simulink model "Senorless"  (R2023a)
settings: Solver=FixedStepDiscrete  StartTime=0.0  StopTime=5  FixedStep=1/FOC_FRQ  RelTol=1e-3
values from neighbouring files (symbols this model uses):
  ADC_REF = 3.6    [Senorless.sldd]
  ADC_SAMPLE_MAX = 32767.0    [Senorless.sldd]
  AMP_GAIN = 16.0    [Senorless.sldd]
  CURR_INPUT = 3276.0    [Senorless.sldd]
  CURR_KI = 380.0    [Senorless.sldd]
  CURR_KP = 0.04    [Senorless.sldd]
  CURR_LIMIT = 0.95    [Senorless.sldd]
  CURR_OVER = 6.0    [Senorless.sldd]
  CURR_POINT_GAIN = 7.0    [Senorless.sldd]
  CURR_STEP = 32760.0    [Senorless.sldd]
  CURR_UNDER = 0.03    [Senorless.sldd]
  CURR_WIDTH = 6552.0    [Senorless.sldd]
  FOC_FRQ = 25000.0    [Senorless.sldd]
  GAMMA = 32767.0    [Senorless.sldd]
  IMAX = 10.0    [Senorless.sldd]
  LPF_FRQ = 2000.0    [Senorless.sldd]
  MOTOR_DAMPER = 2.06E-7    [Senorless.sldd]
  MOTOR_FLUX = 0.00212352    [Senorless.sldd]
  MOTOR_INERTIA = 4.0E-7    [Senorless.sldd]
  MOTOR_LS = 0.000536    [Senorless.sldd]
  MOTOR_PN = 7.0    [Senorless.sldd]
  MOTOR_RS = 4.0    [Senorless.sldd]
  OPEN_IQ = 0.28    [Senorless.sldd]
  OPEN_IQ_MIN = 0.05    [Senorless.sldd]
  OPEN_IQ_SLOW = 0.1    [Senorless.sldd]
  OPEN_SPD = 1000.0    [Senorless.sldd]
  OPEN_SPD_SLOW = 180.0    [Senorless.sldd]
  OPEN_TIME = 0.5    [Senorless.sldd]
  OPEN_TIME_NFO = 0.5    [Senorless.sldd]
  PLL_LIMIT = 0.9    [Senorless.sldd]
  PLL_WIDTH = 800.0    [Senorless.sldd]
  PWM_FRQ = 96000000.0    [Senorless.sldd]
  RS_HUNT = 0.02    [Senorless.sldd]
  SMOK_FRQ = 600.0    [Senorless.sldd]
  SPD_LIMIT = 0.9    [Senorless.sldd]
  SPD_LPF_LEVEL = 0.0    [Senorless.sldd]
  SPD_MAX = 12000.0    [Senorless.sldd]
  SPD_MIN = 4000.0    [Senorless.sldd]
  SPD_REDUCE = 380.0    [Senorless.sldd]
  SPD_STEP = 6.0    [Senorless.sldd]
  SPD_WIDTH = 20.0    [Senorless.sldd]
  THETA_ERR_LIMIT = 8192.0    [Senorless.sldd]
  TS_POINT_GAIN = 10.0    [Senorless.sldd]
  UDC = 48.0    [Senorless.sldd]
  UDC_GAIN = 21.0    [Senorless.sldd]
  UDC_POINT_GAIN = 10.0    [Senorless.sldd]
undefined symbols (not defined in the file or in its folder): curr_q_ki, curr_q_kp, DiscIntNeverNeededParam, magnitude, PLL_LPF_LEVEL, Udc
libraries: simulink x20, slpidlib x5, mcbcontrolslib x2, mcbplantlib x1, autolibpmsmexterior x1, spspowerguiLib x1
(part 3 of 8)

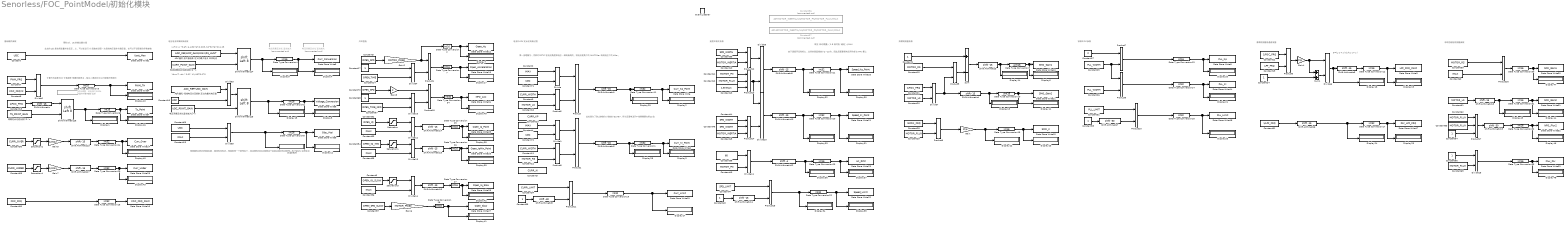
== system Senorless/FOC_PointModel/初始化模块 ==
  note: 非线性磁链观测器参数
  note: 由于速度环没有标幺，出来的是直接放大2^15的，因此后面要把电流环的标幺IMAX算上
  note: 带宽*转动惯量/（1.5*极对数*磁链）/IMAX
  note: 速度环相关系数
  note: 滑模观测器低通滤波器
  note: 锁相环PID参数
  note: 观测器电流电压转换系数，指将电压电流转换到同一个参考系下，如这里电压定点值乘这个后就会换去电流参考：32768/10这种定点
  note: 滑模观测器系数
  note: 开环强拖
  note: 电流环KPKI定点化转换过程
  note: 基础硬件参数
  note: 电压电流采集转换系数
  note: 此处的Udc是全局变量并非宏定义，可以在运行init函数前读取一次母线电压值作为确定值，也可以不读取修改字典参数
  note: 此处是为了防止参数为小数放大32767，所以后面电流环PI结果需要左移15位
  note: 第一部理解为，同样的32767在电流角度和电压角度是不一样的概念，这里是做转换用的，将电流视角下的MAX=IMax转到电压下的UMax。
  note: 限制Ud、Uq的输出最大值
  note: iwf = iw *3.6f / 6.4/32767/0.005 /10*32767=11.25
  note: Vbus = vdc * 3.6f * 41/48=3.075
  note: 计算方式就是PWM计数频率/想要的频率/2，除以二是因为中心计数模式导致的
  note: a=(ω c​ T s​ )/(1+ω c​ T s​ )
  ADC量程*母线电压分压倍数/定义的最大电压值 : Constant  Value=ADC_REF*UDC_GAIN
  ADC量程/放大器倍数/定义的最大电流/采样电流 : Constant  Value=ADC_REF/AMP_GAIN/IMAX/RS_HUNT
  Constant{,69,71..72} (4 alike) : Constant  Value=UDC  OutDataTypeStr=int16
  Constant{1,17,24,33,35,48,68} (7 alike) : Constant  OutDataTypeStr=single
  Constant10 : Constant  Value=MOTOR_LS  OutDataTypeStr=single
  Constant11 : Constant  Value=CURR_WIDTH  OutDataTypeStr=single
  Constant12 : Constant  Value=MOTOR_RS  OutDataTypeStr=single
  Constant13 : Constant  Value=IMAX  OutDataTypeStr=single
  Constant14 : Constant  Value=OPEN_TIME
  Constant15 : Constant  Value=MOTOR_RS  OutDataTypeStr=single
  Constant16 : Constant  Value=UDC
  Constant18 : Constant  Value=1/FOC_FRQ  VectorParams1D=off  OutDataTypeStr=double
  Constant19 : Constant  Value=LPF_FRQ
  Constant2 : Constant  Value=IMAX  OutDataTypeStr=single
  Constant20 : Constant  Value=MOTOR_LS  OutDataTypeStr=single
  Constant21 : Constant  Value=1/FOC_FRQ  VectorParams1D=off  OutDataTypeStr=double
  Constant22 : Constant  Value=1/FOC_FRQ  VectorParams1D=off  OutDataTypeStr=double
  Constant23 : Constant  Value=CURR_KP  OutDataTypeStr=single
  Constant25 : Constant  Value=PLL_WIDTH
  Constant26 : Constant  Value=PLL_WIDTH
  Constant27 : Constant  Value=2  OutDataTypeStr=single
  Constant28 : Constant  Value=SMOK_FRQ
  Constant{29,42,62..63,65} (5 alike) : Constant  Value=MOTOR_FLUX
  Constant3 : Constant  Value=CURR_KI  OutDataTypeStr=single
  Constant30 : Constant  Value=FOC_FRQ  VectorParams1D=off
  Constant31 : Constant  Value=1/LPF_FRQ  VectorParams1D=off  OutDataTypeStr=single
  Constant32 : Constant  Value=PLL_LIMIT
  Constant34 : Constant  Value=CURR_LIMIT  OutDataTypeStr=single
  Constant36 : Constant  Commented=on  Value=40*MOTOR_INERTIA/1.5/MOTOR_PN/MOTOR_FLUX/IMAX  OutDataTypeStr=single
  Constant37 : Constant  Commented=on  Value=40*40*MOTOR_INERTIA/1.5/MOTOR_PN/MOTOR_FLUX/IMAX  OutDataTypeStr=single
  Constant38 : Constant  Value=60  OutDataTypeStr=single
  Constant39 : Constant  Value=SPD_WIDTH
  Constant4 : Constant  Value=IMAX  OutDataTypeStr=single
  Constant40 : Constant  Value=MOTOR_INERTIA
  Constant41 : Constant  Value=MOTOR_PN
  Constant43 : Constant  Value=1.5*IMAX
  Constant44 : Constant  Value=SPD_WIDTH
  Constant45 : Constant  Value=MOTOR_INERTIA
  Constant46 : Constant  Value=SPD_WIDTH
  Constant47 : Constant  Value=SPD_LIMIT
  Constant49 : Constant  Value=MOTOR_PN
  Constant5 : Constant  Value=OPEN_SPD  OutDataTypeStr=single
  Constant50 : Constant  Value=CURR_OVER  VectorParams1D=off
  Constant52 : Constant  Value=OPEN_IQ
  Constant{53,55..56,60} (4 alike) : Constant  Value=IMAX
  Constant54 : Constant  Value=OPEN_IQ_MIN
  Constant57 : Constant  Value=OPEN_SPD_SLOW  OutDataTypeStr=single
  Constant58 : Constant  Value=CURR_UNDER  VectorParams1D=off
  Constant59 : Constant  Value=MOTOR_RS  OutDataTypeStr=single
  Constant6 : Constant  Value=OPEN_IQ_SLOW
  Constant61 : Constant  Value=MOTOR_LS  OutDataTypeStr=single
  Constant64 : Constant
  Constant66 : Constant
  Constant67 : Constant  Value=OPEN_TIME_NFO
  Constant7 : Constant  Value=PWM_FRQ
  Constant70 : Constant  Value=OPEN_SPD  OutDataTypeStr=single
  Constant8 : Constant  Value=FOC_FRQ*2  OutDataTypeStr=double
  Constant9 : Constant  Value=CURR_WIDTH  OutDataTypeStr=single
  Data Store Write : DataStoreWrite  DataStoreName=Curr_Kp_Point  IndexOptions=Index vector (dialog)  Indices=1  OutputSizes=1
  Data Store Write1 : DataStoreWrite  DataStoreName=Uout_Max  IndexOptions=Index vector (dialog)  Indices=1  OutputSizes=1
  Data Store Write10 : DataStoreWrite  DataStoreName=SMO_Gain1  IndexOptions=Index vector (dialog)  Indices=1  OutputSizes=1
  Data Store Write11 : DataStoreWrite  DataStoreName=SMO_Gain2  IndexOptions=Index vector (dialog)  Indices=1  OutputSizes=1
  Data Store Write12 : DataStoreWrite  DataStoreName=Open_Hz  IndexOptions=Index vector (dialog)  Indices=1  OutputSizes=1
  Data Store Write13 : DataStoreWrite  DataStoreName=Open_Acceleration  IndexOptions=Index vector (dialog)  Indices=1  OutputSizes=1
  Data Store Write14 : DataStoreWrite  DataStoreName=PLL_Ki  IndexOptions=Index vector (dialog)  Indices=1  OutputSizes=1
  Data Store Write15 : DataStoreWrite  DataStoreName=SMO_K  IndexOptions=Index vector (dialog)  Indices=1  OutputSizes=1
  Data Store Write16 : DataStoreWrite  DataStoreName=FOC_FRQ_Point  IndexOptions=Index vector (dialog)  Indices=1  OutputSizes=1
  Data Store Write17 : DataStoreWrite  DataStoreName=DIV_LPF_FRQ  IndexOptions=Index vector (dialog)  Indices=1  OutputSizes=1
  Data Store Write18 : DataStoreWrite  DataStoreName=PLL_Limit  IndexOptions=Index vector (dialog)  Indices=1  OutputSizes=1
  Data Store Write19 : DataStoreWrite  DataStoreName=Curr_Limit  IndexOptions=Index vector (dialog)  Indices=1  OutputSizes=1
  Data Store Write2 : DataStoreWrite  DataStoreName=Curr_Ki_Point  IndexOptions=Index vector (dialog)  Indices=1  OutputSizes=1
  Data Store Write20 : DataStoreWrite  DataStoreName=Speed_Kp_Point  IndexOptions=Index vector (dialog)  Indices=1  OutputSizes=1
  Data Store Write21 : DataStoreWrite  DataStoreName=Speed_Ki_Point  IndexOptions=Index vector (dialog)  Indices=1  OutputSizes=1
  Data Store Write22 : DataStoreWrite  DataStoreName=Speed_Limit  IndexOptions=Index vector (dialog)  Indices=1  OutputSizes=1
  Data Store Write23 : DataStoreWrite  DataStoreName=Hz_RPM  IndexOptions=Index vector (dialog)  Indices=1  OutputSizes=1
  Data Store Write24 : DataStoreWrite  DataStoreName=Curr_Over  IndexOptions=Index vector (dialog)  Indices=1  OutputSizes=1
  Data Store Write25 : DataStoreWrite  DataStoreName=Open_Iq_Point  IndexOptions=Index vector (dialog)  Indices=1  OutputSizes=1
  Data Store Write26 : DataStoreWrite  DataStoreName=Open_IqMin_Point  IndexOptions=Index vector (dialog)  Indices=1  OutputSizes=1
  Data Store Write27 : DataStoreWrite  DataStoreName=Open_Slow  IndexOptions=Index vector (dialog)  Indices=1  OutputSizes=1
  Data Store Write28 : DataStoreWrite  DataStoreName=Open_Iq_Slow  IndexOptions=Index vector (dialog)  Indices=1  OutputSizes=1
  Data Store Write29 : DataStoreWrite  DataStoreName=Curr_Under  IndexOptions=Index vector (dialog)  Indices=1  OutputSizes=1
  Data Store Write3 : DataStoreWrite  DataStoreName=LPF_FRQ_Point  IndexOptions=Index vector (dialog)  Indices=1  OutputSizes=1
  Data Store Write30 : DataStoreWrite  DataStoreName=NFO_Gain1  IndexOptions=Index vector (dialog)  Indices=1  OutputSizes=1
  Data Store Write31 : DataStoreWrite  DataStoreName=NFO_Gain2  IndexOptions=Index vector (dialog)  Indices=1  OutputSizes=1
  Data Store Write32 : DataStoreWrite  DataStoreName=NFO_Flux2  IndexOptions=Index vector (dialog)  Indices=1  OutputSizes=1
  Data Store Write33 : DataStoreWrite  DataStoreName=Flux_Div  IndexOptions=Index vector (dialog)  Indices=1  OutputSizes=1
  Data Store Write34 : DataStoreWrite  DataStoreName=NFO_Acc  IndexOptions=Index vector (dialog)  Indices=1  OutputSizes=1
  Data Store Write4 : DataStoreWrite  DataStoreName=PWM_TH  IndexOptions=Index vector (dialog)  Indices=1  OutputSizes=1
  Data Store Write5 : DataStoreWrite  DataStoreName=Curr_Conversion  IndexOptions=Index vector (dialog)  Indices=1  OutputSizes=1
  Data Store Write6 : DataStoreWrite  DataStoreName=Voltage_Conversion  IndexOptions=Index vector (dialog)  Indices=1  OutputSizes=1
  Data Store Write7 : DataStoreWrite  Priority=-1  DataStoreName=Ts_Point  IndexOptions=Index vector (dialog)  Indices=1  OutputSizes=1
  Data Store Write8 : DataStoreWrite  DataStoreName=PLL_Kp  IndexOptions=Index vector (dialog)  Indices=1  OutputSizes=1
  Data Store Write9 : DataStoreWrite  DataStoreName=Obs_VtoI  IndexOptions=Index vector (dialog)  Indices=1  OutputSizes=1
  Data Type Conversion{1,11,14,16..19,22,24,29,34} (11 alike) : DataTypeConversion  OutDataTypeStr=int32  RndMeth=Nearest  SaturateOnIntegerOverflow=off
  Data Type Conversion10 : DataTypeConversion  OutDataTypeStr=uint16  RndMeth=Nearest  SaturateOnIntegerOverflow=off
  Data Type Conversion{12,15,23,30..33} (7 alike) : DataTypeConversion  OutDataTypeStr=int16  RndMeth=Ceiling  SaturateOnIntegerOverflow=off
  Data Type Conversion{2..8,13,25..28} (12 alike) : DataTypeConversion  OutDataTypeStr=int16  RndMeth=Nearest  SaturateOnIntegerOverflow=off
  Data Type Conversion20 : DataTypeConversion  OutDataTypeStr=int32  RndMeth=Ceiling  SaturateOnIntegerOverflow=off
  Data Type Conversion21 : DataTypeConversion  OutDataTypeStr=int32  RndMeth=Ceiling  SaturateOnIntegerOverflow=off
  Data Type Conversion9 : DataTypeConversion  OutDataTypeStr=uint16  RndMeth=Nearest  SaturateOnIntegerOverflow=off
  Display{1..49} (49 alike) : Display
  Divide{,1..2,4..7,9,11..16} (14 alike) : Product  Inputs=*/
  Divide10 : Product  Inputs=/*
  Divide3 : Product  Inputs=*/  RndMeth=Zero
  Event Listener : EventListener  DisableCoverage=on  EventName=reset
  Gain : Gain  Gain=2*pi
  Gain2 : Gain  Gain=MOTOR_PN/60
  Gain4 : Gain  Gain=2*pi
  Gain5 : Gain  Gain=1/IMAX
  Gain6 : Gain  Gain=MOTOR_PN/60
  Gain7 : Gain  Gain=1/IMAX
  Gain8 : Gain  Gain=2
  Product{,1..12,15..16,18} (16 alike) : Product
  Product13 : Product  Inputs=3
  Product14 : Product  Inputs=3
  Product17 : Product  Inputs=3
  Saturation{,1..4} (5 alike) : Saturate  UpperLimit=IMAX  LowerLimit=-IMAX
  Shift Arithmetic{,1..6,9..11,13..18} (16 alike) : ArithShift  BitShiftNumber=-15
  Shift Arithmetic12 : ArithShift  BitShiftNumber=-4
  Shift Arithmetic19 : ArithShift  BitShiftNumber=-30
  Shift Arithmetic24 : ArithShift  BitShiftNumberSource=Input port  BitShiftNumber=8  BitShiftDirection=Left
      settings: InputPortMap=u0,p1
  Shift Arithmetic25 : ArithShift  BitShiftNumberSource=Input port  BitShiftNumber=8  BitShiftDirection=Left
      settings: InputPortMap=u0,p1
  Shift Arithmetic26 : ArithShift  BitShiftNumberSource=Input port  BitShiftNumber=8  BitShiftDirection=Left
      settings: InputPortMap=u0,p1
  Shift Arithmetic7 : ArithShift  BitShiftNumber=-30
  Shift Arithmetic8 : ArithShift  BitShiftNumber=-30
  Sum : Sum  Inputs=+-
  Sum1 : Sum
  周期定点化适当放大2^n : Constant  Value=TS_POINT_GAIN
  电压采集定点化 适当放大 : ArithShift  Commented=on  BitShiftNumber=-UDC_POINT_GAIN  DiagnosticForOORShift=Error
  电压采集定点化适当放大2^n : Constant  Value=UDC_POINT_GAIN
  电流采集定点化 适当放大 : ArithShift  Commented=on  BitShiftNumber=-CURR_POINT_GAIN  DiagnosticForOORShift=Error
  电流采集定点化适当放大2^n : Constant  Value=CURR_POINT_GAIN
  适当调整，此处放大1024 : ArithShift  Commented=on  BitShiftNumber=-TS_POINT_GAIN  DiagnosticForOORShift=Error
  wires:
  Product/1 -> Shift Arithmetic1/1
  Constant2/1 -> Divide/1
  Constant71/1 -> Divide/2
  Divide/1 -> Product/1
  Data Type Conversion11/1 -> Display2/1, Data Store Write/1
  Constant/1 -> Data Store Write1/1
  Constant9/1 -> Product2/1
  Constant10/1 -> Product2/2
  Data Type Conversion4/1 -> Display4/1, Data Store Write5/1
  ADC量程/放大器倍数/定义的最大电流/采样电流/1 -> Shift Arithmetic24/1
  Shift Arithmetic24/1 -> Display9/1, Data Type Conversion4/1
  Data Type Conversion5/1 -> Display5/1, Data Store Write6/1
  ADC量程*母线电压分压倍数/定义的最大电压值/1 -> Divide3/1
  Constant16/1 -> Divide3/2
  Divide3/1 -> Shift Arithmetic25/1
  Shift Arithmetic1/1 -> Display29/1, Data Type Conversion11/1
  Constant14/1 -> Divide4/2
  Constant17/1 -> Divide4/1
  Constant5/1 -> Gain2/1
  Gain2/1 -> Data Type Conversion2/1, Product4/1
  Data Type Conversion2/1 -> Display7/1, Data Store Write12/1
  Product4/1 -> Data Type Conversion7/1
  Divide4/1 -> Product4/2
  Data Type Conversion8/1 -> Display12/1, Data Store Write9/1
  Data Type Conversion3/1 -> Display10/1, Data Store Write4/1
  Data Type Conversion6/1 -> Display16/1, Data Store Write7/1
  Constant7/1 -> Divide2/1
  Shift Arithmetic/1 -> Shift Arithmetic26/1
  Constant18/1 -> Shift Arithmetic/1
  Divide2/1 -> Data Type Conversion3/1
  Shift Arithmetic26/1 -> Display1/1, Data Type Conversion6/1
  Constant8/1 -> Divide2/2
  Data Type Conversion9/1 -> Display6/1, Data Store Write10/1
  Divide5/1 -> Display8/1, Data Type Conversion8/1
  Constant69/1 -> Divide5/1
  Constant13/1 -> Divide5/2
  Constant21/1 -> Divide7/1
  Constant20/1 -> Divide7/2
  Divide7/1 -> Product5/2, Shift Arithmetic4/1
  Shift Arithmetic2/1 -> Display28/1, Data Type Conversion1/1
  Constant12/1 -> Product3/2
  Constant11/1 -> Product3/1
  Product1/1 -> Shift Arithmetic2/1
  Divide1/1 -> Product1/1
  Constant4/1 -> Divide1/1
  Constant72/1 -> Divide1/2
  Data Type Conversion1/1 -> Display3/1, Data Store Write2/1
  Shift Arithmetic25/1 -> Data Type Conversion5/1, Display15/1
  Data Type Conversion10/1 -> Display11/1, Data Store Write11/1
  Shift Arithmetic3/1 -> Display14/1, Data Type Conversion9/1
  Shift Arithmetic4/1 -> Display13/1, Data Type Conversion10/1
  Sum/1 -> Shift Arithmetic3/1
  Constant1/1 -> Sum/1
  Product5/1 -> Sum/2
  Constant15/1 -> Product5/1
  Data Type Conversion12/1 -> Display19/1, Data Store Write3/1
  Shift Arithmetic5/1 -> Data Type Conversion12/1
  Constant22/1 -> Product6/1
  Constant19/1 -> Product6/2
  Sum1/1 -> Divide6/2
  Constant24/1 -> Sum1/2
  Divide6/1 -> Display18/1, Shift Arithmetic5/1
  Constant25/1 -> Product8/1, Product7/2
  Constant27/1 -> Product7/1
  Constant26/1 -> Product8/2
  Product7/1 -> Data Type Conversion13/1
  Product8/1 -> Data Type Conversion14/1
  Data Type Conversion13/1 -> Display20/1, Data Store Write8/1
  Data Type Conversion14/1 -> Display21/1, Data Store Write14/1
  Constant28/1 -> Product9/1
  Constant29/1 -> Product9/2
  Gain/1 -> Data Type Conversion15/1, Display22/1
  Data Type Conversion15/1 -> Data Store Write15/1, Display23/1
  Data Type Conversion16/1 -> Data Store Write16/1
  Constant30/1 -> Data Type Conversion16/1
  Product2/1 -> Product/2
  Product3/1 -> Product1/2
  Shift Arithmetic6/1 -> Display24/1, Data Type Conversion17/1
  Constant31/1 -> Shift Arithmetic6/1
  Data Type Conversion17/1 -> Display25/1, Data Store Write17/1
  电流采集定点化适当放大2^n/1 -> Shift Arithmetic24/2
  电压采集定点化适当放大2^n/1 -> Shift Arithmetic25/2
  周期定点化适当放大2^n/1 -> Shift Arithmetic26/2
  Constant32/1 -> Product10/1
  Constant33/1 -> Shift Arithmetic7/1
  Shift Arithmetic7/1 -> Product10/2
  Product10/1 -> Data Type Conversion18/1
  Data Type Conversion18/1 -> Display26/1, Data Store Write18/1
  Shift Arithmetic8/1 -> Product11/2
  Constant34/1 -> Product11/1
  Constant35/1 -> Shift Arithmetic8/1
  Product11/1 -> Data Type Conversion19/1
  Data Type Conversion19/1 -> Display27/1, Data Store Write19/1
  Product9/1 -> Gain/1
  Shift Arithmetic10/1 -> Data Type Conversion20/1, Display33/1
  Shift Arithmetic9/1 -> Data Type Conversion21/1, Display32/1
  Constant39/1 -> Product12/1
  Constant40/1 -> Product12/2
  Constant42/1 -> Product13/2
  Constant43/1 -> Product13/3
  Product12/1 -> Divide9/1
  Product13/1 -> Divide10/1, Divide9/2
  Constant44/1 -> Product14/1
  Constant45/1 -> Product14/3
  Constant46/1 -> Product14/2
  Product14/1 -> Divide10/2
  Divide9/1 -> Shift Arithmetic9/1
  Divide10/1 -> Shift Arithmetic10/1
  Data Type Conversion21/1 -> Display30/1, Data Store Write20/1
  Data Type Conversion20/1 -> Display31/1, Data Store Write21/1
  Product15/1 -> Display34/1, Data Type Conversion22/1
  Shift Arithmetic11/1 -> Product15/2
  Constant47/1 -> Product15/1
  Constant48/1 -> Shift Arithmetic11/1
  Data Type Conversion22/1 -> Data Store Write22/1, Display35/1
  Constant41/1 -> Product13/1
  Divide11/1 -> Shift Arithmetic12/1
  Shift Arithmetic12/1 -> Display36/1, Data Type Conversion23/1
  Data Type Conversion23/1 -> Display37/1, Data Store Write23/1
  Constant49/1 -> Divide11/2
  Constant38/1 -> Divide11/1
  Constant50/1 -> Saturation2/1
  Shift Arithmetic13/1 -> Data Type Conversion24/1
  Data Type Conversion24/1 -> Display40/1, Data Store Write24/1
  Product6/1 -> Gain4/1
  Gain4/1 -> Sum1/1, Divide6/1
  Constant52/1 -> Saturation/1
  Saturation/1 -> Divide12/1
  Constant53/1 -> Divide12/2
  Divide12/1 -> Shift Arithmetic14/1
  Shift Arithmetic14/1 -> Data Type Conversion25/1
  Constant54/1 -> Saturation1/1
  Constant55/1 -> Divide13/2
  Divide13/1 -> Shift Arithmetic15/1
  Shift Arithmetic15/1 -> Data Type Conversion26/1
  Data Type Conversion25/1 -> Data Store Write25/1, Display38/1
  Data Type Conversion26/1 -> Display39/1, Data Store Write26/1
  Saturation1/1 -> Divide13/1
  Saturation2/1 -> Gain5/1
  Gain5/1 -> Shift Arithmetic13/1
  Shift Arithmetic16/1 -> Data Type Conversion27/1
  Constant56/1 -> Divide14/2
  Constant6/1 -> Saturation3/1
  Divide14/1 -> Shift Arithmetic16/1
  Saturation3/1 -> Divide14/1
  Gain6/1 -> Data Type Conversion28/1
  Data Type Conversion28/1 -> Data Store Write27/1, Display41/1
  Constant57/1 -> Gain6/1
  Data Type Conversion7/1 -> Display17/1, Data Store Write13/1
  Data Type Conversion27/1 -> Display42/1, Data Store Write28/1
  Data Type Conversion29/1 -> Display43/1, Data Store Write29/1
  Shift Arithmetic17/1 -> Data Type Conversion29/1
  Gain7/1 -> Shift Arithmetic17/1
  Saturation4/1 -> Gain7/1
  Constant58/1 -> Saturation4/1
  Product16/1 -> Data Type Conversion30/1
  Data Type Conversion30/1 -> Display47/1, Data Store Write30/1
  Constant59/1 -> Product16/1
  Constant60/1 -> Product16/2
  Data Type Conversion31/1 -> Display44/1, Data Store Write31/1
  Shift Arithmetic18/1 -> Data Type Conversion31/1, Display45/1
  Constant61/1 -> Shift Arithmetic18/1
  Constant62/1 -> Product17/1
  Product17/1 -> Shift Arithmetic19/1
  Shift Arithmetic19/1 -> Data Type Conversion32/1
  Data Type Conversion32/1 -> Display46/1, Data Store Write32/1
  Constant63/1 -> Product17/2
  Constant64/1 -> Product17/3
  Constant65/1 -> Divide15/2
  Constant66/1 -> Divide15/1
  Divide15/1 -> Data Type Conversion33/1
  Data Type Conversion33/1 -> Display48/1, Data Store Write33/1
  Constant67/1 -> Divide16/2
  Divide16/1 -> Product18/2
  Constant68/1 -> Divide16/1
  Constant70/1 -> Gain8/1
  Data Type Conversion34/1 -> Display49/1, Data Store Write34/1
  Product18/1 -> Data Type Conversion34/1
  Gain8/1 -> Product18/1

== system Senorless/FOC_PointModel/加速强拖 ==
  Acc : Inport  OutDataTypeStr=int16  PortDimensions=1
  Action Port : ActionPort  InitializeStates=reset  ActionPortLabel=case [ 2 ]:
  Constant1 : Constant  Value=0  OutDataTypeStr=int16
  Data Store Read3 : DataStoreRead  DataStoreName=Open_Iq_Point  IndexOptions=Index vector (dialog)  Indices=1  OutputSizes=1
  FreqGenerator_point2 : Subsystem  Commented=on
  Subsystem : Subsystem  Commented=on
  加速积分角度 : Subsystem
  Theta : Outport
  Iq : Outport  Port=2
  Id : Outport  Port=3
  wires:
  Acc/1 -> 加速积分角度/1(Acc)
  加速积分角度/1(Theta) -> Theta/1
  Constant1/1 -> Id/1
  Data Store Read3/1 -> Iq/1

== system Senorless/FOC_PointModel/恒速降力矩强拖 ==
  Hz : Inport  OutDataTypeStr=int16  PortDimensions=1
  Xo : Inport  Port=2
  Action Port : ActionPort  InitializeStates=reset  ActionPortLabel=case [ 3 ]:
  Bias : Bias  Bias=int16(1)  SaturateOnIntegerOverflow=off
  Constant1 : Constant  Commented=on  OutDataTypeStr=int16
  Constant2 : Constant  Commented=on  Value=0  OutDataTypeStr=int16
  Constant3 : Constant  Commented=on  Value=0  OutDataTypeStr=int16
  Constant7 : Constant  Value=0  OutDataTypeStr=int16
  Constant8 : Constant  Value=0  OutDataTypeStr=int16
  Data Store Read1 : DataStoreRead  DataStoreName=Open_IqMin_Point  IndexOptions=Index vector (dialog)  Indices=1  OutputSizes=1
  Data Store Read2 : DataStoreRead  DataStoreName=Open_Iq_Point  IndexOptions=Index vector (dialog)  Indices=1  OutputSizes=1
  Data Store Read3 : DataStoreRead  DataStoreName=Open_Iq_Point  IndexOptions=Index vector (dialog)  Indices=1  OutputSizes=1
  Data Type Conversion : DataTypeConversion  OutDataTypeStr=uint16  SaturateOnIntegerOverflow=off
  Data Type Conversion1 : DataTypeConversion  OutDataTypeStr=int32  SaturateOnIntegerOverflow=off
  Data Type Conversion2 : DataTypeConversion  OutDataTypeStr=int32  SaturateOnIntegerOverflow=off
  FreqGenerator_point2 : Subsystem  Commented=on
  MATLAB Function : MATLAB Function  Commented=on  TreatAsAtomicUnit=on
  Saturation Dynamic2 : simulink/Discontinuities/Saturation Dynamic  OutMin=[]  OutMax=[]  OutDataTypeStr=Inherit: Same as second input  OutDataType=fixdt(1, 16)  OutScaling=2^-10  RndMeth=Zero  DoSatur=off
  Saturation2 : Saturate  Commented=on  UpperLimit=0  LowerLimit=-3276  RndMeth=Zero
  Scope1 : Scope  NumInputPorts=2
  Shift Arithmetic : ArithShift  BitShiftNumber=-16
  Sum : Sum  Inputs=|+-
  Sum1 : Sum  Inputs=|+-
  Sum3 : Sum  Commented=on  Inputs=|-+
  Unit Delay1 : UnitDelay  SampleTime=-1  HasFrameUpgradeWarning=on
  Unit Delay2 : UnitDelay  Commented=on  SampleTime=-1  HasFrameUpgradeWarning=on
  积分器 : Subsystem
      settings: MinAlgLoopOccurrences=on
  Theta : Outport
  Iq : Outport  Port=2
  Id : Outport  Port=3
  wires:
  Constant2/1 -> MATLAB Function/2(u2)
  Data Store Read2/1 -> Sum1/1
  Saturation2/1 -> Unit Delay2/1
  Unit Delay2/1 -> Sum3/2
  Sum3/1 -> Saturation2/1
  Constant1/1 -> Sum3/1
  Data Type Conversion/1 -> Scope1/2, Theta/1
  Sum1/1 -> Iq/1
  Saturation Dynamic2/1 -> Unit Delay1/1
  Bias/1 -> Saturation Dynamic2/2
  Unit Delay1/1 -> Sum1/2, Bias/1, Id/1
  Sum/1 -> Saturation Dynamic2/1
  Data Store Read3/1 -> Sum/1
  Data Store Read1/1 -> Sum/2
  Constant7/1 -> Saturation Dynamic2/3
  Data Type Conversion1/1 -> 积分器/2(Xo)
  Xo/1 -> Data Type Conversion1/1
  Hz/1 -> Data Type Conversion2/1
  Data Type Conversion2/1 -> Shift Arithmetic/1
  Shift Arithmetic/1 -> 积分器/1(input)
  积分器/1(output) -> Scope1/1, Data Type Conversion/1

== system Senorless/FOC_PointModel/慢速开环 ==
  Hz : Inport  OutDataTypeStr=int16  PortDimensions=1
  Action Port : ActionPort  InitializeStates=reset  ActionPortLabel=case [ 5 ]:
  Constant8 : Constant  Value=0  OutDataTypeStr=int16
  Data Store Read6 : DataStoreRead  DataStoreName=Open_Iq_Slow  IndexOptions=Index vector (dialog)  Indices=1  OutputSizes=1
  Data Type Conversion : DataTypeConversion  OutDataTypeStr=uint16  SaturateOnIntegerOverflow=off
  Data Type Conversion2 : DataTypeConversion  OutDataTypeStr=int32  SaturateOnIntegerOverflow=off
  FreqGenerator_point2 : Subsystem  Commented=on
  Scope1 : Scope  NumInputPorts=2
  Shift Arithmetic : ArithShift  BitShiftNumber=-16
  积分器 : Subsystem
      settings: MinAlgLoopOccurrences=on
  Theta : Outport
  Iq : Outport  Port=2
  Id : Outport  Port=3
  wires:
  Constant8/1 -> Id/1
  Data Type Conversion/1 -> Theta/1, Scope1/2
  Data Store Read6/1 -> Iq/1
  积分器/1(output) -> Scope1/1, Data Type Conversion/1
  Shift Arithmetic/1 -> 积分器/1(input)
  Data Type Conversion2/1 -> Shift Arithmetic/1
  Hz/1 -> Data Type Conversion2/1

== system Senorless/FOC_PointModel/电压限转速 ==
  note: 通过实时检测母线电压，调整最大转速
  Udc_Ref : Inport
  SPD_Ref : Inport  Port=2
  Constant1 : Constant  Value=SPD_REDUCE  OutDataTypeStr=int32
  Constant2 : Constant  Value=0  OutDataTypeStr=int32
  Constant4 : Constant  Value=UDC  OutDataTypeStr=int16
  Constant5 : Constant  Value=UDC-6  OutDataTypeStr=int16
  Constant6 : Constant  Value=SPD_MAX  OutDataTypeStr=int32
  Constant7 : Constant  Value=SPD_MIN  OutDataTypeStr=int32
  Product : Product  OutDataTypeStr=int32  RndMeth=Zero
  Product4 : Product  OutDataTypeStr=int32
  Saturation : Saturate  UpperLimit=UDC  LowerLimit=0
  Saturation Dynamic2 : simulink/Discontinuities/Saturation Dynamic  OutMin=[]  OutMax=[]  OutDataTypeStr=Inherit: Same as second input  OutDataType=fixdt(1, 16)  OutScaling=2^-10  RndMeth=Zero  DoSatur=off
  Shift Arithmetic : ArithShift  BitShiftNumber=15
  Sum : Sum  Inputs=-+  OutDataTypeStr=int16  RndMeth=Zero
  Sum2 : Sum  Inputs=+-  RndMeth=Zero
  out : Outport
  wires:
  Constant5/1 -> Sum/2
  Product4/1 -> Shift Arithmetic/1
  Constant4/1 -> Product4/1
  Sum/1 -> Saturation/1
  Shift Arithmetic/1 -> Sum/1
  SPD_Ref/1 -> Saturation Dynamic2/2
  Udc_Ref/1 -> Product4/2
  Sum2/1 -> Saturation Dynamic2/1
  Saturation Dynamic2/1 -> out/1
  Constant7/1 -> Saturation Dynamic2/3
  Constant1/1 -> Product/1
  Saturation/1 -> Product/2
  Constant6/1 -> Sum2/1
  Product/1 -> Sum2/2

== system Senorless/FOC_PointModel/积分器 ==
  input : Inport
  Constant : Constant  OutDataTypeStr=int16
  Data Store Read1 : DataStoreRead  DataStoreName=Ts_Point  IndexOptions=Index vector (dialog)  Indices=1  OutputSizes=1
  Product1 : Product  OutDataTypeStr=int32  RndMeth=Zero
  Product2 : Product  OutDataTypeStr=int32  RndMeth=Zero
  Shift Arithmetic : ArithShift  BitShiftNumberSource=Input port  BitShiftNumber=8  BitShiftDirection=Right
      settings: InputPortMap=u0,p1
  Sum : Sum  Inputs=|++  OutDataTypeStr=int32  RndMeth=Zero
  Unit Delay : UnitDelay  SampleTime=-1  HasFrameUpgradeWarning=on
  周期定点化适当放大2^n : Constant  Value=TS_POINT_GAIN
  这个是缩小周期增益的 : ArithShift  BitShiftNumber=15  DiagnosticForOORShift=Error
  output : Outport
  wires:
  周期定点化适当放大2^n/1 -> Shift Arithmetic/2
  Shift Arithmetic/1 -> Product2/2
  Data Store Read1/1 -> Product2/1
  input/1 -> Shift Arithmetic/1
  这个是缩小周期增益的/1 -> Product1/2
  Product2/1 -> 这个是缩小周期增益的/1
  Product1/1 -> Sum/1
  Sum/1 -> Unit Delay/1, output/1
  Unit Delay/1 -> Sum/2
  Constant/1 -> Product1/1

== system Senorless/FOC_PointModel/积分器1 ==
  input : Inport
  Constant : Constant  OutDataTypeStr=int16
  Data Store Read1 : DataStoreRead  DataStoreName=Ts_Point  IndexOptions=Index vector (dialog)  Indices=1  OutputSizes=1
  Product1 : Product  OutDataTypeStr=int32  RndMeth=Zero
  Product2 : Product  OutDataTypeStr=int32  RndMeth=Zero
  Shift Arithmetic : ArithShift  BitShiftNumberSource=Input port  BitShiftNumber=8  BitShiftDirection=Right
      settings: InputPortMap=u0,p1
  Sum : Sum  Inputs=|++  OutDataTypeStr=int32  RndMeth=Zero
  Unit Delay : UnitDelay  SampleTime=-1  HasFrameUpgradeWarning=on
  周期定点化适当放大2^n : Constant  Value=TS_POINT_GAIN
  这个是缩小周期增益的 : ArithShift  BitShiftNumber=15  DiagnosticForOORShift=Error
  output : Outport
  wires:
  Constant/1 -> Product1/1
  Unit Delay/1 -> Sum/2
  Sum/1 -> output/1, Unit Delay/1
  Product1/1 -> Sum/1
  Product2/1 -> 这个是缩小周期增益的/1
  这个是缩小周期增益的/1 -> Product1/2
  input/1 -> Shift Arithmetic/1
  Data Store Read1/1 -> Product2/1
  Shift Arithmetic/1 -> Product2/2
  周期定点化适当放大2^n/1 -> Shift Arithmetic/2

== system Senorless/FOC_PointModel/积分器2 ==
  input : Inport
  Constant : Constant  OutDataTypeStr=int16
  Data Store Read1 : DataStoreRead  DataStoreName=Ts_Point  IndexOptions=Index vector (dialog)  Indices=1  OutputSizes=1
  Product1 : Product  OutDataTypeStr=int32  RndMeth=Zero
  Product2 : Product  OutDataTypeStr=int32  RndMeth=Zero
  Shift Arithmetic : ArithShift  BitShiftNumberSource=Input port  BitShiftNumber=8  BitShiftDirection=Right
      settings: InputPortMap=u0,p1
  Sum : Sum  Inputs=|++  OutDataTypeStr=int32  RndMeth=Zero
  Unit Delay : UnitDelay  SampleTime=-1  HasFrameUpgradeWarning=on
  周期定点化适当放大2^n : Constant  Value=TS_POINT_GAIN
  这个是缩小周期增益的 : ArithShift  BitShiftNumber=15  DiagnosticForOORShift=Error
  output : Outport
  wires:
  Constant/1 -> Product1/1
  Unit Delay/1 -> Sum/2
  Sum/1 -> output/1, Unit Delay/1
  Product1/1 -> Sum/1
  Product2/1 -> 这个是缩小周期增益的/1
  这个是缩小周期增益的/1 -> Product1/2
  input/1 -> Shift Arithmetic/1
  Data Store Read1/1 -> Product2/1
  Shift Arithmetic/1 -> Product2/2
  周期定点化适当放大2^n/1 -> Shift Arithmetic/2

== system Senorless/FOC_PointModel/积分器3 ==
  input : Inport
  Constant : Constant  OutDataTypeStr=int16
  Data Store Read1 : DataStoreRead  DataStoreName=Ts_Point  IndexOptions=Index vector (dialog)  Indices=1  OutputSizes=1
  Product1 : Product  OutDataTypeStr=int32  RndMeth=Zero
  Product2 : Product  OutDataTypeStr=int32  RndMeth=Zero
  Shift Arithmetic : ArithShift  BitShiftNumberSource=Input port  BitShiftNumber=8  BitShiftDirection=Right
      settings: InputPortMap=u0,p1
  Sum : Sum  Inputs=|++  OutDataTypeStr=int32  RndMeth=Zero
  Unit Delay : UnitDelay  SampleTime=-1  HasFrameUpgradeWarning=on
  周期定点化适当放大2^n : Constant  Value=TS_POINT_GAIN
  这个是缩小周期增益的 : ArithShift  BitShiftNumber=15  DiagnosticForOORShift=Error
  output : Outport
  wires:
  周期定点化适当放大2^n/1 -> Shift Arithmetic/2
  Shift Arithmetic/1 -> Product2/2
  Data Store Read1/1 -> Product2/1
  input/1 -> Shift Arithmetic/1
  这个是缩小周期增益的/1 -> Product1/2
  Product2/1 -> 这个是缩小周期增益的/1
  Product1/1 -> Sum/1
  Sum/1 -> Unit Delay/1, output/1
  Unit Delay/1 -> Sum/2
  Constant/1 -> Product1/1

== system Senorless/FOC_PointModel/积分器4 ==
  input : Inport
  Constant : Constant  OutDataTypeStr=int16
  Data Store Read1 : DataStoreRead  DataStoreName=Ts_Point  IndexOptions=Index vector (dialog)  Indices=1  OutputSizes=1
  Product1 : Product  OutDataTypeStr=int32  RndMeth=Zero
  Product2 : Product  OutDataTypeStr=int32  RndMeth=Zero
  Shift Arithmetic : ArithShift  BitShiftNumberSource=Input port  BitShiftNumber=8  BitShiftDirection=Right
      settings: InputPortMap=u0,p1
  Sum : Sum  Inputs=|++  OutDataTypeStr=int32  RndMeth=Zero
  Unit Delay : UnitDelay  SampleTime=-1  HasFrameUpgradeWarning=on
  周期定点化适当放大2^n : Constant  Value=TS_POINT_GAIN
  这个是缩小周期增益的 : ArithShift  BitShiftNumber=15  DiagnosticForOORShift=Error
  output : Outport
  wires:
  Constant/1 -> Product1/1
  Unit Delay/1 -> Sum/2
  Sum/1 -> output/1, Unit Delay/1
  Product1/1 -> Sum/1
  Product2/1 -> 这个是缩小周期增益的/1
  这个是缩小周期增益的/1 -> Product1/2
  input/1 -> Shift Arithmetic/1
  Data Store Read1/1 -> Product2/1
  Shift Arithmetic/1 -> Product2/2
  周期定点化适当放大2^n/1 -> Shift Arithmetic/2

== system Senorless/FOC_PointModel/积分器5 ==
  input : Inport
  Constant : Constant  OutDataTypeStr=int16
  Data Store Read1 : DataStoreRead  DataStoreName=Ts_Point  IndexOptions=Index vector (dialog)  Indices=1  OutputSizes=1
  Product1 : Product  OutDataTypeStr=int32  RndMeth=Zero
  Product2 : Product  OutDataTypeStr=int32  RndMeth=Zero
  Shift Arithmetic : ArithShift  BitShiftNumberSource=Input port  BitShiftNumber=8  BitShiftDirection=Right
      settings: InputPortMap=u0,p1
  Sum : Sum  Inputs=|++  OutDataTypeStr=int32  RndMeth=Zero
  Unit Delay : UnitDelay  SampleTime=-1  HasFrameUpgradeWarning=on
  周期定点化适当放大2^n : Constant  Value=TS_POINT_GAIN
  这个是缩小周期增益的 : ArithShift  BitShiftNumber=15  DiagnosticForOORShift=Error
  output : Outport
  wires:
  周期定点化适当放大2^n/1 -> Shift Arithmetic/2
  Shift Arithmetic/1 -> Product2/2
  Data Store Read1/1 -> Product2/1
  input/1 -> Shift Arithmetic/1
  这个是缩小周期增益的/1 -> Product1/2
  Product2/1 -> 这个是缩小周期增益的/1
  Product1/1 -> Sum/1
  Sum/1 -> Unit Delay/1, output/1
  Unit Delay/1 -> Sum/2
  Constant/1 -> Product1/1
